simulink model "canrx_0x14FFBF17"  (R2022b)
settings: configuration reference "SLDD_CFG" (kept outside this file)
values from neighbouring files (symbols this model uses):
  D_DRV_RETARDER_REQ_MAX = 1.0    [canrx_0x14FFBF17.sldd]
  D_DRV_RETARDER_REQ_MIN = 0.0    [canrx_0x14FFBF17.sldd]
  K_CAN_GMLAN_RX_INVALID_SELECT = 0.0    [canrx_0x14FFBF17.sldd]
  K_CAN_J1939_RX_DEFAULT_DRV_RETARDER_REQ = 0.0    [canrx_0x14FFBF17.sldd]
  PLCANC_APCNTL_RQST_SEL_GMLAN = 1.0    [canrx_0x14FFBF17.sldd]
  PLCANC_APCNTL_RQST_SEL_J1939 = 0.0    [canrx_0x14FFBF17.sldd]
libraries: user_lib x1, simulink x1
settings Model: DataDictionary=canrx_0x14FFBF17.sldd  Creator=Castiel  LastModifiedBy=Castiel
settings ConfigSetRef: SourceName=SLDD_CFG

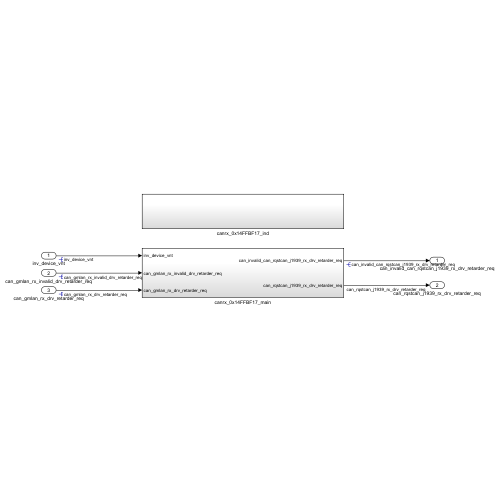
[thumbnail: Simulink's stored preview of the top-level diagram]
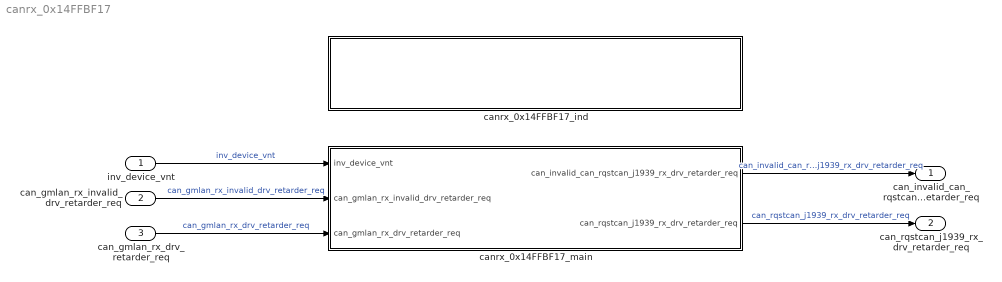
== system canrx_0x14FFBF17 ==
  inv_device_vnt : Inport
  can_gmlan_rx_invalid_drv_retarder_req : Inport  Port=2
  can_gmlan_rx_drv_retarder_req : Inport  Port=3
  canrx_0x14FFBF17_ind : Subsystem
  canrx_0x14FFBF17_main : Subsystem
  can_invalid_can_rqstcan_j1939_rx_drv_retarder_req : Outport
  can_rqstcan_j1939_rx_drv_retarder_req : Outport  Port=2
  wires:
  inv_device_vnt/1 -> canrx_0x14FFBF17_main/1(inv_device_vnt)  "inv_device_vnt"
  can_gmlan_rx_invalid_drv_retarder_req/1 -> canrx_0x14FFBF17_main/2(can_gmlan_rx_invalid_drv_retarder_req)  "can_gmlan_rx_invalid_drv_retarder_req"
  can_gmlan_rx_drv_retarder_req/1 -> canrx_0x14FFBF17_main/3(can_gmlan_rx_drv_retarder_req)  "can_gmlan_rx_drv_retarder_req"
  canrx_0x14FFBF17_main/1(can_invalid_can_rqstcan_j1939_rx_drv_retarder_req) -> can_invalid_can_rqstcan_j1939_rx_drv_retarder_req/1  "can_invalid_can_rqstcan_j1939_rx_drv_retarder_req"
  canrx_0x14FFBF17_main/2(can_rqstcan_j1939_rx_drv_retarder_req) -> can_rqstcan_j1939_rx_drv_retarder_req/1  "can_rqstcan_j1939_rx_drv_retarder_req"

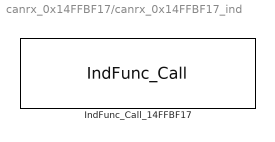
== system canrx_0x14FFBF17/canrx_0x14FFBF17_ind ==
  IndFunc_Call_14FFBF17 : user_lib/IndFunc_Call  siggroupIndex=Test  canid=14FFBF17  signalTable={'UB','IFLayer_can_j1939_rx_drv_retarder_req','SYCANC_COM2AP_14FFBF17_can_j1939_rx_drv_retarder_req'}  timeoutflag=on  extendid=on
      settings: SourceProductName=User Defined for IFLayer

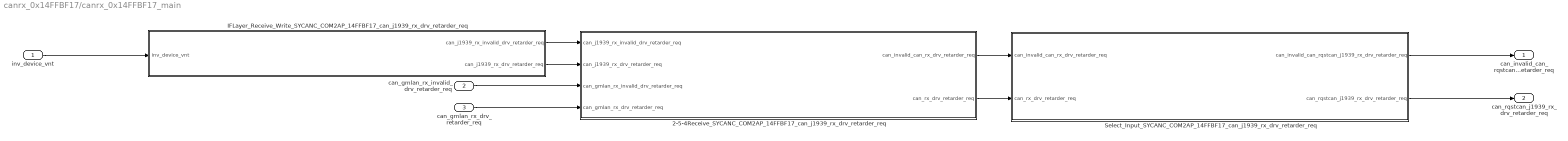
== system canrx_0x14FFBF17/canrx_0x14FFBF17_main ==
  inv_device_vnt : Inport
  can_gmlan_rx_invalid_drv_retarder_req : Inport  Port=2
  can_gmlan_rx_drv_retarder_req : Inport  Port=3
  2-5-4Receive_SYCANC_COM2AP_14FFBF17_can_j1939_rx_drv_retarder_req : Subsystem  TreatAsAtomicUnit=on
      settings: RTWSystemCode=Nonreusable function
  IFLayer_Receive_Write_SYCANC_COM2AP_14FFBF17_can_j1939_rx_drv_retarder_req : Subsystem  TreatAsAtomicUnit=on
      settings: RTWSystemCode=Nonreusable function
  Select_Input_SYCANC_COM2AP_14FFBF17_can_j1939_rx_drv_retarder_req : Subsystem  TreatAsAtomicUnit=on
      settings: RTWSystemCode=Nonreusable function
  can_invalid_can_rqstcan_j1939_rx_drv_retarder_req : Outport
  can_rqstcan_j1939_rx_drv_retarder_req : Outport  Port=2
  wires:
  IFLayer_Receive_Write_SYCANC_COM2AP_14FFBF17_can_j1939_rx_drv_retarder_req/2(can_j1939_rx_drv_retarder_req) -> 2-5-4Receive_SYCANC_COM2AP_14FFBF17_can_j1939_rx_drv_retarder_req/2(can_j1939_rx_drv_retarder_req)
  IFLayer_Receive_Write_SYCANC_COM2AP_14FFBF17_can_j1939_rx_drv_retarder_req/1(can_j1939_rx_invalid_drv_retarder_req) -> 2-5-4Receive_SYCANC_COM2AP_14FFBF17_can_j1939_rx_drv_retarder_req/1(can_j1939_rx_invalid_drv_retarder_req)
  2-5-4Receive_SYCANC_COM2AP_14FFBF17_can_j1939_rx_drv_retarder_req/1(can_invalid_can_rx_drv_retarder_req) -> Select_Input_SYCANC_COM2AP_14FFBF17_can_j1939_rx_drv_retarder_req/1(can_invalid_can_rx_drv_retarder_req)
  2-5-4Receive_SYCANC_COM2AP_14FFBF17_can_j1939_rx_drv_retarder_req/2(can_rx_drv_retarder_req) -> Select_Input_SYCANC_COM2AP_14FFBF17_can_j1939_rx_drv_retarder_req/2(can_rx_drv_retarder_req)
  inv_device_vnt/1 -> IFLayer_Receive_Write_SYCANC_COM2AP_14FFBF17_can_j1939_rx_drv_retarder_req/1(inv_device_vnt)
  can_gmlan_rx_invalid_drv_retarder_req/1 -> 2-5-4Receive_SYCANC_COM2AP_14FFBF17_can_j1939_rx_drv_retarder_req/3(can_gmlan_rx_invalid_drv_retarder_req)
  can_gmlan_rx_drv_retarder_req/1 -> 2-5-4Receive_SYCANC_COM2AP_14FFBF17_can_j1939_rx_drv_retarder_req/4(can_gmlan_rx_drv_retarder_req)
  Select_Input_SYCANC_COM2AP_14FFBF17_can_j1939_rx_drv_retarder_req/1(can_invalid_can_rqstcan_j1939_rx_drv_retarder_req) -> can_invalid_can_rqstcan_j1939_rx_drv_retarder_req/1
  Select_Input_SYCANC_COM2AP_14FFBF17_can_j1939_rx_drv_retarder_req/2(can_rqstcan_j1939_rx_drv_retarder_req) -> can_rqstcan_j1939_rx_drv_retarder_req/1

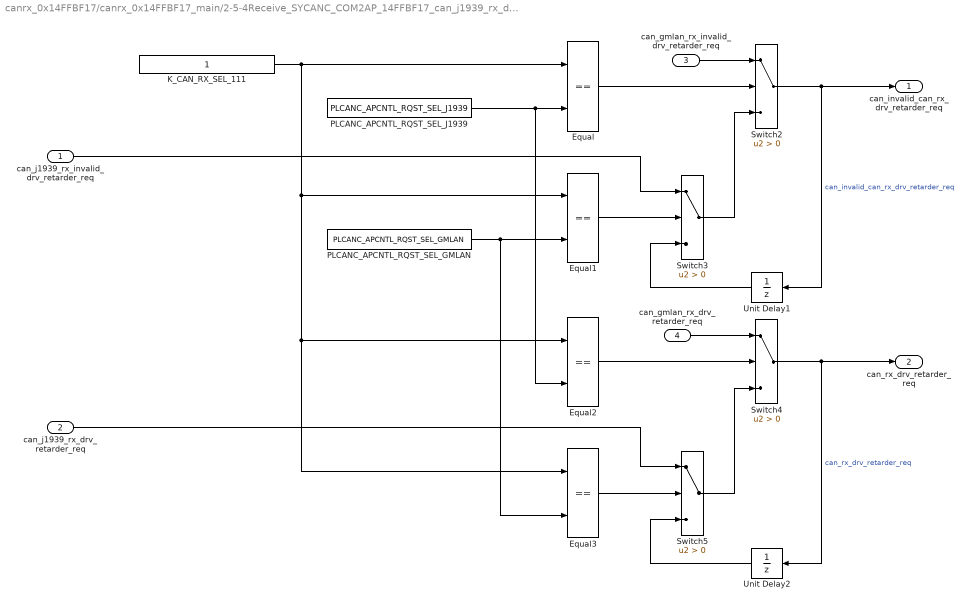
== system canrx_0x14FFBF17/canrx_0x14FFBF17_main/2-5-4Receive_SYCANC_COM2AP_14FFBF17_can_j1939_rx_drv_retarder_req ==
  can_j1939_rx_invalid_drv_retarder_req : Inport
  can_j1939_rx_drv_retarder_req : Inport  Port=2
  can_gmlan_rx_invalid_drv_retarder_req : Inport  Port=3
  can_gmlan_rx_drv_retarder_req : Inport  Port=4
  Equal{,1..3} (4 alike) : RelationalOperator  Operator===  OutDataTypeStr=boolean  RndMeth=Simplest  InputSameDT=off
  K_CAN_RX_SEL_111 : Constant
  PLCANC_APCNTL_RQST_SEL_GMLAN : Constant  Value=PLCANC_APCNTL_RQST_SEL_GMLAN
  PLCANC_APCNTL_RQST_SEL_J1939 : Constant  Value=PLCANC_APCNTL_RQST_SEL_J1939
  Switch{2..5} (4 alike) : Switch  Criteria=u2 > Threshold  SaturateOnIntegerOverflow=off  InputSameDT=off
  Unit Delay1 : UnitDelay  SampleTime=-1  HasFrameUpgradeWarning=on
  Unit Delay2 : UnitDelay  SampleTime=-1  HasFrameUpgradeWarning=on
  can_invalid_can_rx_drv_retarder_req : Outport
  can_rx_drv_retarder_req : Outport  Port=2
  wires:
  Switch3/1 -> Switch2/3
  can_gmlan_rx_drv_retarder_req/1 -> Switch4/1
  K_CAN_RX_SEL_111/1 -> Equal/1, Equal1/1, Equal2/1, Equal3/1
  Switch4/1 -> can_rx_drv_retarder_req/1, Unit Delay2/1  "can_rx_drv_retarder_req"
  PLCANC_APCNTL_RQST_SEL_J1939/1 -> Equal/2, Equal2/2
  can_j1939_rx_drv_retarder_req/1 -> Switch5/1
  Equal2/1 -> Switch4/2
  can_gmlan_rx_invalid_drv_retarder_req/1 -> Switch2/1
  PLCANC_APCNTL_RQST_SEL_GMLAN/1 -> Equal1/2, Equal3/2
  can_j1939_rx_invalid_drv_retarder_req/1 -> Switch3/1
  Switch5/1 -> Switch4/3
  Equal3/1 -> Switch5/2
  Equal1/1 -> Switch3/2
  Unit Delay2/1 -> Switch5/3
  Switch2/1 -> can_invalid_can_rx_drv_retarder_req/1, Unit Delay1/1  "can_invalid_can_rx_drv_retarder_req"
  Unit Delay1/1 -> Switch3/3
  Equal/1 -> Switch2/2

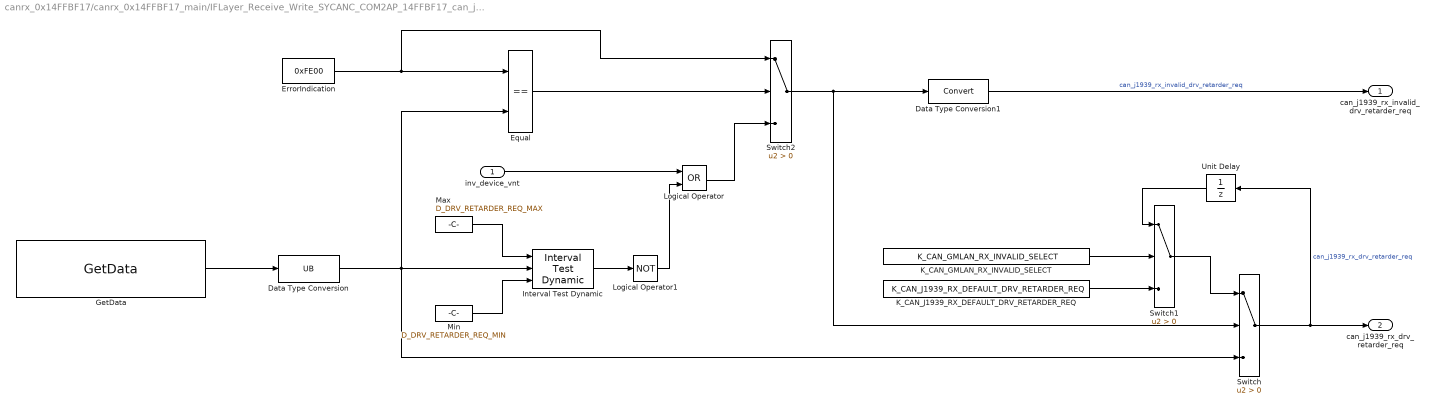
== system canrx_0x14FFBF17/canrx_0x14FFBF17_main/IFLayer_Receive_Write_SYCANC_COM2AP_14FFBF17_can_j1939_rx_drv_retarder_req ==
  inv_device_vnt : Inport
  Data Type Conversion : DataTypeConversion  OutDataTypeStr=UB  ConvertRealWorld=Stored Integer (SI)  SaturateOnIntegerOverflow=off  RndMeth=Floor
  Data Type Conversion1 : DataTypeConversion  ConvertRealWorld=Stored Integer (SI)  SaturateOnIntegerOverflow=off  RndMeth=Floor
  Equal : RelationalOperator  Operator===  OutDataTypeStr=boolean  RndMeth=Simplest  InputSameDT=off
  ErrorIndication : Constant  Value=0xFE00  OutDataTypeStr=Inherit: Inherit via back propagation
  GetData : S-Function  FunctionName=GetData  Parameters=interface,signalType  SFunctionDeploymentMode=off  EnableBusSupport=off  mask{interface=SYCANC_COM2AP_14FFBF17_can_j1939_rx_drv_retarder_req, signalType=UB}
      mask prompts: signalType "Signal Type"
      mask TypeOptions signalType: UB | SB | UW | SW | UD | SD
      mask DialogControl Container4 Prompt: Singal Parameter
      mask Display:
      | interfaceName = get_param(gcbh, "interface");
      | s = strcat(interfaceName);
      | disp(s);
  Interval Test Dynamic : simulink/Logic and Bit Operations/Interval Test Dynamic  IntervalClosedRight=on  IntervalClosedLeft=on  OutDataTypeStr=boolean
  K_CAN_GMLAN_RX_INVALID_SELECT : Constant  Value=K_CAN_GMLAN_RX_INVALID_SELECT  OutDataTypeStr=Inherit: Inherit via back propagation
  K_CAN_J1939_RX_DEFAULT_DRV_RETARDER_REQ : Constant  Value=K_CAN_J1939_RX_DEFAULT_DRV_RETARDER_REQ  OutDataTypeStr=Inherit: Inherit via back propagation
  Logical Operator : Logic  Operator=OR  AllPortsSameDT=off  OutDataTypeStr=boolean
  Logical Operator1 : Logic  Operator=NOT  AllPortsSameDT=off  OutDataTypeStr=boolean
  Max : Constant  Value=D_DRV_RETARDER_REQ_MAX  OutDataTypeStr=Inherit: Inherit via back propagation
  Min : Constant  Value=D_DRV_RETARDER_REQ_MIN  OutDataTypeStr=Inherit: Inherit via back propagation
  Switch : Switch  Criteria=u2 > Threshold  SaturateOnIntegerOverflow=off  InputSameDT=off
  Switch1 : Switch  Criteria=u2 > Threshold  SaturateOnIntegerOverflow=off  InputSameDT=off
  Switch2 : Switch  Criteria=u2 > Threshold  SaturateOnIntegerOverflow=off  InputSameDT=off
  Unit Delay : UnitDelay  SampleTime=-1  HasFrameUpgradeWarning=on
  can_j1939_rx_invalid_drv_retarder_req : Outport
  can_j1939_rx_drv_retarder_req : Outport  Port=2
  wires:
  Switch1/1 -> Switch/1
  Unit Delay/1 -> Switch1/1
  inv_device_vnt/1 -> Logical Operator/1
  K_CAN_J1939_RX_DEFAULT_DRV_RETARDER_REQ/1 -> Switch1/3
  Max/1 -> Interval Test Dynamic/1
  Min/1 -> Interval Test Dynamic/3
  Switch/1 -> Unit Delay/1, can_j1939_rx_drv_retarder_req/1  "can_j1939_rx_drv_retarder_req"
  K_CAN_GMLAN_RX_INVALID_SELECT/1 -> Switch1/2
  Data Type Conversion1/1 -> can_j1939_rx_invalid_drv_retarder_req/1  "can_j1939_rx_invalid_drv_retarder_req"
  Logical Operator1/1 -> Logical Operator/2
  Interval Test Dynamic/1 -> Logical Operator1/1
  GetData/1 -> Data Type Conversion/1
  Switch2/1 -> Switch/2, Data Type Conversion1/1
  Equal/1 -> Switch2/2
  Logical Operator/1 -> Switch2/3
  Data Type Conversion/1 -> Equal/2, Switch/3, Interval Test Dynamic/2
  ErrorIndication/1 -> Switch2/1, Equal/1

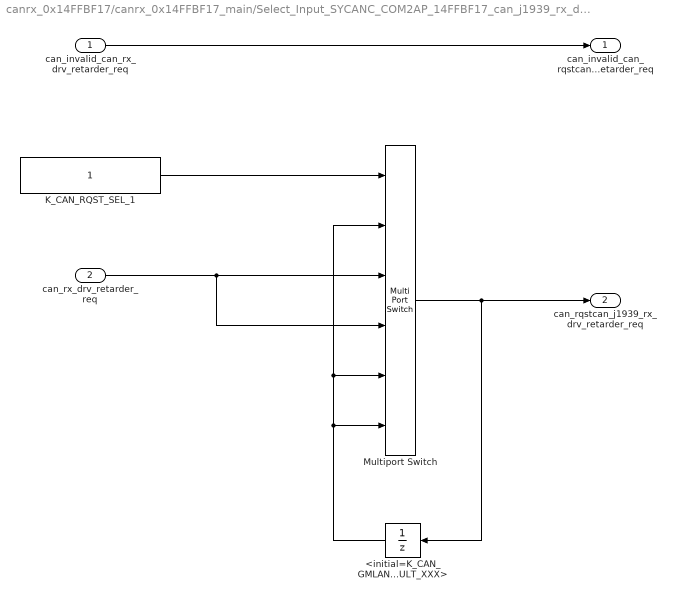
== system canrx_0x14FFBF17/canrx_0x14FFBF17_main/Select_Input_SYCANC_COM2AP_14FFBF17_can_j1939_rx_drv_retarder_req ==
  can_invalid_can_rx_drv_retarder_req : Inport
  can_rx_drv_retarder_req : Inport  Port=2
  <initial=K_CAN_GMLAN_RX_DEFAULT_XXX> : UnitDelay  SampleTime=-1  HasFrameUpgradeWarning=on
  K_CAN_RQST_SEL_1 : Constant
  Multiport Switch : MultiPortSwitch  DataPortOrder=Zero-based contiguous  Inputs=5  zeroidx=on  SaturateOnIntegerOverflow=off  InputSameDT=off
  can_invalid_can_rqstcan_j1939_rx_drv_retarder_req : Outport
  can_rqstcan_j1939_rx_drv_retarder_req : Outport  Port=2
  wires:
  K_CAN_RQST_SEL_1/1 -> Multiport Switch/1
  <initial=K_CAN_GMLAN_RX_DEFAULT_XXX>/1 -> Multiport Switch/6, Multiport Switch/2, Multiport Switch/5
  Multiport Switch/1 -> can_rqstcan_j1939_rx_drv_retarder_req/1, <initial=K_CAN_GMLAN_RX_DEFAULT_XXX>/1
  can_rx_drv_retarder_req/1 -> Multiport Switch/4, Multiport Switch/3
  can_invalid_can_rx_drv_retarder_req/1 -> can_invalid_can_rqstcan_j1939_rx_drv_retarder_req/1
